simulink model "tp1_simulink"  (R2020a)
settings: Solver=VariableStepAuto  StartTime=0.0  StopTime=10.0  RelTol=1e-3
settings Model: Creator=Usuario  LastModifiedBy=Usuario

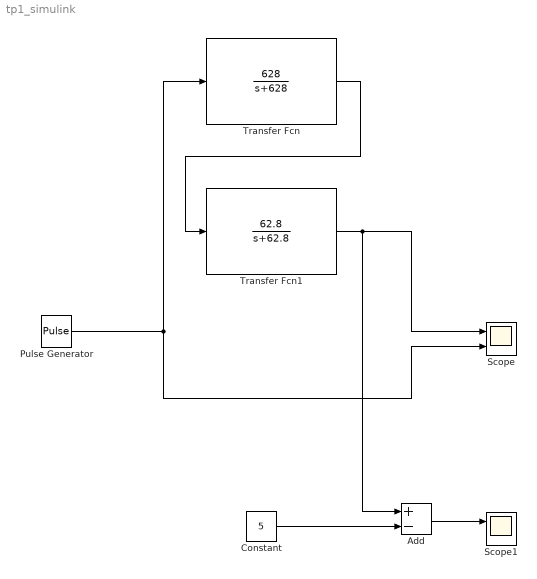
== system tp1_simulink ==
  Add : Sum  Inputs=+-
  Constant : Constant  Value=5
  Pulse Generator : DiscretePulseGenerator  PulseType=Time based  Amplitude=10  Period=0.001  PulseWidth=50
  Scope : Scope  NumInputPorts=2
  Scope1 : Scope  NumInputPorts=2
  Transfer Fcn : TransferFcn  Numerator=[628]  Denominator=[1 628]
  Transfer Fcn1 : TransferFcn  Numerator=[62.8]  Denominator=[1 62.8]
  wires:
  Pulse Generator/1 -> Scope/2, Transfer Fcn/1
  Add/1 -> Scope1/1
  Constant/1 -> Add/2
  Transfer Fcn/1 -> Transfer Fcn1/1
  Transfer Fcn1/1 -> Add/1, Scope/1
